simulink model "f_cd_reorder"  (R2018a)
settings: Solver=VariableStepAuto  StartTime=0.0  StopTime=200000  RelTol=1e-3
libraries: xbsIndex_r4 x1711, casper_library_misc x12, xps_library x2, simulink x1
(part 1 of 9)
settings Model: Creator=andrew  LastModifiedBy=andrew

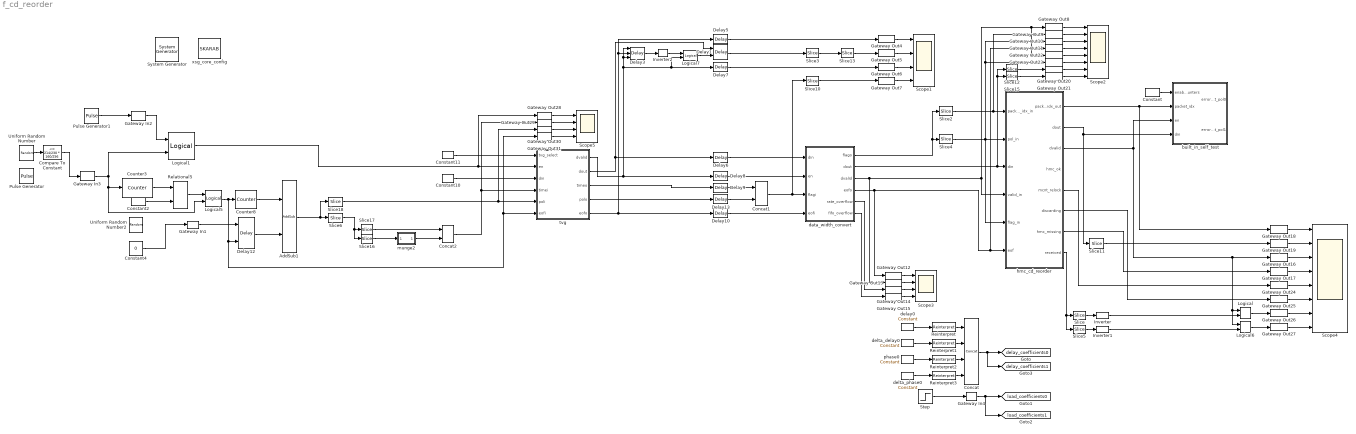
== system f_cd_reorder ==
  " System Generator" : xbsIndex_r4/ System Generator  Tag=genX  xilinxfamily=virtex7  part=xc7vx690t  speed=-2  package=ffg1927  synthesis_tool=XST  clock_wrapper=Clock Enables  directory=/home/skarab_fpga/source/feng_wide/s_c856m1k/sysgen  proj_type=Vivado  Synth_file=Vivado Synthesis Defaults  Impl_file=Vivado Implementation Defaults  testbench=off  simulink_period=1  sysclk_period=4.2017  dcm_input_clock_period=10  incr_netlist=off  trim_vbits=Everywhere in SubSystem  dbl_ovrd=According to Block Masks  core_generation=According to Block Masks  run_coregen=off  deprecated_control=off  eval_field=0  block_type=sysgen
  AddSub1 : xbsIndex_r4/AddSub  mode=Addition  use_carryin=off  use_carryout=off  en=off  latency=0  precision=User Defined  arith_type=Unsigned  n_bits=36+1  bin_pt=0  quantization=Truncate  overflow=Wrap  use_behavioral_HDL=off  hw_selection=Fabric  pipelined=off  dbl_ovrd=off  block_type=addsub
  Compare To Constant : simulink/Logic and Bit Operations/Compare To Constant  relop=<=  const=214/230 * 160/256  OutDataTypeStr=boolean
  Concat : xbsIndex_r4/Concat  num_inputs=4  dbl_ovrd=off  block_type=concat
  Concat1 : xbsIndex_r4/Concat  num_inputs=2  dbl_ovrd=off  block_type=concat
  Concat2 : xbsIndex_r4/Concat  num_inputs=2  dbl_ovrd=off  block_type=concat
  Constant : xbsIndex_r4/Constant  const=1  gui_display_data_type=Boolean  arith_type=Boolean  n_bits=1  bin_pt=0  preci_type=Single  exp_width=8  frac_width=24  explicit_period=on  period=1  equ=P=C  opselect=C  inp2=PCIN>>17  opr=+  inp1=P  carry=CIN  dbl_ovrd=off  block_type=constant
  Constant10 : xbsIndex_r4/Constant  const=0  gui_display_data_type=Fixed-point  arith_type=Unsigned  n_bits=256  bin_pt=0  preci_type=Single  exp_width=8  frac_width=24  explicit_period=on  period=1  equ=P=C  opselect=C  inp2=PCIN>>17  opr=+  inp1=P  carry=CIN  dbl_ovrd=off  block_type=constant
  Constant11 : xbsIndex_r4/Constant  const=1  gui_display_data_type=Fixed-point  arith_type=Unsigned  n_bits=1  bin_pt=0  preci_type=Single  exp_width=8  frac_width=24  explicit_period=on  period=1  equ=P=C  opselect=C  inp2=PCIN>>17  opr=+  inp1=P  carry=CIN  dbl_ovrd=off  block_type=constant
  Constant2 : xbsIndex_r4/Constant  const=(4096*10)/256-1  gui_display_data_type=Fixed-point  arith_type=Unsigned  n_bits=ceil(log2((4096*10)/256))  bin_pt=0  preci_type=Single  exp_width=8  frac_width=24  explicit_period=on  period=1  equ=P=C  opselect=C  inp2=PCIN>>17  opr=+  inp1=P  carry=CIN  dbl_ovrd=off  block_type=constant
  Constant4 : Constant  Value=0
  Counter3 : xbsIndex_r4/Counter  cnt_type=Count Limited  cnt_to=((4096*10)/256)-1  operation=Up  start_count=0  cnt_by_val=1  arith_type=Unsigned  n_bits=ceil(log2((4096*10)/256))  bin_pt=0  load_pin=off  rst=off  en=on  explicit_period=on  period=1  use_behavioral_HDL=off  implementation=Fabric  dbl_ovrd=off  block_type=counter
  Counter8 : xbsIndex_r4/Counter  cnt_type=Free Running  cnt_to=48  operation=Up  start_count=0*167  cnt_by_val=1  arith_type=Unsigned  n_bits=36+1  bin_pt=0  load_pin=off  rst=off  en=on  explicit_period=on  period=1  use_behavioral_HDL=off  implementation=Fabric  dbl_ovrd=off  block_type=counter
  Delay1 : xbsIndex_r4/Delay  rst=off  infoeditControl=Selection of Reset will increase slice count due to use of real FFs and instead of SRLs  en=on  latency=1  reg_retiming=on  dbl_ovrd=off  block_type=delay
  Delay{5..10,13} (7 alike) : xbsIndex_r4/Delay  rst=off  infoeditControl=Selection of Reset will increase slice count due to use of real FFs and instead of SRLs  en=off  latency=1  reg_retiming=on  dbl_ovrd=off  block_type=delay
  Delay12 : xbsIndex_r4/Delay  rst=off  infoeditControl=Selection of Reset will increase slice count due to use of real FFs and instead of SRLs  en=on  latency=1  reg_retiming=off  dbl_ovrd=off  block_type=delay
  Delay3 : xbsIndex_r4/Delay  rst=on  infoeditControl=Selection of Reset will increase slice count due to use of real FFs and instead of SRLs  en=on  latency=1  reg_retiming=on  dbl_ovrd=off  block_type=delay
  Gateway In1 : xbsIndex_r4/Gateway In  gui_display_data_type=Fixed-point  arith_type="Signed  (2's comp)"  n_bits=9  bin_pt=0  preci_type=Single  exp_width=8  frac_width=24  rows=1  columns=1  quantization="Round  (unbiased: +/- Inf)"  overflow=Saturate  period=1  UseAsADC=off  ADCChannel='1'  interface=None  automatic_assignment=on  address_offset=hex2dec('00')  intf_name=''  intf_description=''  default_value=0  timing_constraint=None  locs_specified=off  LOCs={}  io_standard={}  inherit_from_input=off  hdl_port=on  dbl_ovrd=off  block_type=gatewayin
  Gateway In2 : xbsIndex_r4/Gateway In  gui_display_data_type=Boolean  arith_type=Boolean  n_bits=16  bin_pt=14  preci_type=Single  exp_width=8  frac_width=24  rows=1  columns=1  quantization="Round  (unbiased: +/- Inf)"  overflow=Saturate  period=1  UseAsADC=off  ADCChannel='1'  interface=None  automatic_assignment=on  address_offset=hex2dec('00')  intf_name=''  intf_description=''  default_value=0  timing_constraint=None  locs_specified=off  LOCs={}  io_standard={}  inherit_from_input=off  hdl_port=on  dbl_ovrd=off  block_type=gatewayin
  Gateway In3 : xbsIndex_r4/Gateway In  gui_display_data_type=Boolean  arith_type=Boolean  n_bits=16  bin_pt=14  preci_type=Single  exp_width=8  frac_width=24  rows=1  columns=1  quantization="Round  (unbiased: +/- Inf)"  overflow=Saturate  period=1  UseAsADC=off  ADCChannel='1'  interface=None  automatic_assignment=on  address_offset=hex2dec('00')  intf_name=''  intf_description=''  default_value=0  timing_constraint=None  locs_specified=off  LOCs={}  io_standard={}  inherit_from_input=off  hdl_port=on  dbl_ovrd=off  block_type=gatewayin
  Gateway In4 : xbsIndex_r4/Gateway In  gui_display_data_type=Boolean  arith_type=Boolean  n_bits=16  bin_pt=14  preci_type=Single  exp_width=8  frac_width=24  rows=1  columns=1  quantization="Round  (unbiased: +/- Inf)"  overflow=Saturate  period=1  UseAsADC=off  ADCChannel='1'  interface=None  automatic_assignment=on  address_offset=hex2dec('00')  intf_name=''  intf_description=''  default_value=0  timing_constraint=None  locs_specified=off  LOCs={}  io_standard={}  inherit_from_input=off  hdl_port=on  dbl_ovrd=off  block_type=gatewayin
  Gateway Out{4..31} (28 alike) : xbsIndex_r4/Gateway Out  inherit_from_input=off  hdl_port=off  rows=1  columns=1  UseAsDAC=off  DACChannel='1'  interface=None  automatic_assignment=on  address_offset=hex2dec('00')  intf_name=''  intf_description=''  timing_constraint=None  locs_specified=off  LOCs={}  io_standard={}  block_type=gatewayout
  Inverter : xbsIndex_r4/Inverter  en=off  latency=0  dbl_ovrd=off  block_type=inv
  Inverter1 : xbsIndex_r4/Inverter  en=off  latency=0  dbl_ovrd=off  block_type=inv
  Inverter2 : xbsIndex_r4/Inverter  en=off  latency=0  dbl_ovrd=off  block_type=inv
  Logical{,1,5..7} (5 alike) : xbsIndex_r4/Logical  logical_function=AND  inputs=2  en=off  latency=0  precision=Full  arith_type=Unsigned  n_bits=16  bin_pt=0  align_bp=on  dbl_ovrd=off  block_type=logical
  Pulse Generator : DiscretePulseGenerator  Period=floor(256*(240/214))  PulseWidth=160  PhaseDelay=10
  Pulse Generator1 : DiscretePulseGenerator  Period=50000  PulseWidth=45000
  Reinterpret{,1..3} (4 alike) : xbsIndex_r4/Reinterpret  force_arith_type=on  arith_type=Unsigned  force_bin_pt=on  bin_pt=0  block_type=reinterpret
  Relational5 : xbsIndex_r4/Relational  mode=a=b  op_type=Bool  en=off  latency=0  dbl_ovrd=off  block_type=relational
  Scope1 : Scope  NumInputPorts=4
  Scope2 : Scope  NumInputPorts=8
  Scope3 : Scope  NumInputPorts=4
  Scope4 : Scope  NumInputPorts=8
  Scope5 : Scope  NumInputPorts=4
  Slice : xbsIndex_r4/Slice  nbits=1  boolean_output=on  mode=Upper Bit Location + Width  bit1=0  base1=MSB of Input  bit0=0  base0=LSB of Input  dbl_ovrd=off  block_type=slice
  Slice10 : xbsIndex_r4/Slice  nbits=49-12-1  boolean_output=off  mode=Upper Bit Location + Width  bit1=0  base1=MSB of Input  bit0=0  base0=LSB of Input  dbl_ovrd=off  block_type=slice
  Slice11 : xbsIndex_r4/Slice  nbits=80  boolean_output=off  mode=Upper Bit Location + Width  bit1=0  base1=MSB of Input  bit0=0  base0=LSB of Input  dbl_ovrd=off  block_type=slice
  Slice12 : xbsIndex_r4/Slice  nbits=80  boolean_output=off  mode=Upper Bit Location + Width  bit1=0  base1=MSB of Input  bit0=0  base0=LSB of Input  dbl_ovrd=off  block_type=slice
  Slice13 : xbsIndex_r4/Slice  nbits=36  boolean_output=off  mode=Lower Bit Location + Width  bit1=0  base1=MSB of Input  bit0=5+4+1  base0=LSB of Input  dbl_ovrd=off  block_type=slice
  Slice15 : xbsIndex_r4/Slice  nbits=80  boolean_output=off  mode=Lower Bit Location + Width  bit1=0  base1=MSB of Input  bit0=0  base0=LSB of Input  dbl_ovrd=off  block_type=slice
  Slice16 : xbsIndex_r4/Slice  nbits=10  boolean_output=off  mode=Lower Bit Location + Width  bit1=0  base1=MSB of Input  bit0=0  base0=LSB of Input  dbl_ovrd=off  block_type=slice
  Slice17 : xbsIndex_r4/Slice  nbits=8  boolean_output=off  mode=Two Bit Locations  bit1=0  base1=MSB of Input  bit0=10  base0=LSB of Input  dbl_ovrd=off  block_type=slice
  Slice18 : xbsIndex_r4/Slice  nbits=1  boolean_output=off  mode=Lower Bit Location + Width  bit1=0  base1=MSB of Input  bit0=0  base0=LSB of Input  dbl_ovrd=off  block_type=slice
  Slice2 : xbsIndex_r4/Slice  nbits=48-12  boolean_output=off  mode=Upper Bit Location + Width  bit1=0  base1=MSB of Input  bit0=0  base0=LSB of Input  dbl_ovrd=off  block_type=slice
  Slice3 : xbsIndex_r4/Slice  nbits=80  boolean_output=off  mode=Upper Bit Location + Width  bit1=0  base1=MSB of Input  bit0=0  base0=LSB of Input  dbl_ovrd=off  block_type=slice
  Slice4 : xbsIndex_r4/Slice  nbits=1  boolean_output=off  mode=Lower Bit Location + Width  bit1=0  base1=MSB of Input  bit0=0  base0=LSB of Input  dbl_ovrd=off  block_type=slice
  Slice5 : xbsIndex_r4/Slice  nbits=1  boolean_output=on  mode=Lower Bit Location + Width  bit1=0  base1=MSB of Input  bit0=0  base0=LSB of Input  dbl_ovrd=off  block_type=slice
  Slice6 : xbsIndex_r4/Slice  nbits=36  boolean_output=off  mode=Upper Bit Location + Width  bit1=0  base1=MSB of Input  bit0=0  base0=LSB of Input  dbl_ovrd=off  block_type=slice
  Step : Step  SampleTime=300
  Uniform Random Number : UniformRandomNumber  Minimum=0  SampleTime=1
  Uniform Random Number2 : UniformRandomNumber  Minimum=0  SampleTime=1
  built_in_self_test : Subsystem
  data_width_convert : Subsystem  mask{mux_latency=3, n_bits_din=256, n_bits_dout=160, max_burst_len=160*2}
      mask prompts: mux_latency "mux latency"; n_bits_din "data with in"; n_bits_dout "data width out"; max_burst_len "expected max input burst length"
      mask init:
      | %annotation = sprintf('latency=%i', mux_latency);
      | %set_param(gcb, 'AttributesFormatString', annotation);
      | annotation = sprintf('');
      | set_param(gcb, 'AttributesFormatString', annotation);
  delay0 : xbsIndex_r4/Constant  const=0  gui_display_data_type=Fixed-point  arith_type=Unsigned  n_bits=32  bin_pt=15  preci_type=Single  exp_width=8  frac_width=24  explicit_period=on  period=1  equ=P=C  opselect=C  inp2=PCIN>>17  opr=+  inp1=P  carry=CIN  dbl_ovrd=off  block_type=constant
  delta_delay0 : xbsIndex_r4/Constant  const=0  gui_display_data_type=Fixed-point  arith_type=Signed (2's comp)  n_bits=16  bin_pt=15  preci_type=Single  exp_width=8  frac_width=24  explicit_period=on  period=1  equ=P=C  opselect=C  inp2=PCIN>>17  opr=+  inp1=P  carry=CIN  dbl_ovrd=off  block_type=constant
  delta_phase0 : xbsIndex_r4/Constant  const=0  gui_display_data_type=Fixed-point  arith_type=Signed (2's comp)  n_bits=16  bin_pt=15  preci_type=Single  exp_width=8  frac_width=24  explicit_period=on  period=1  equ=P=C  opselect=C  inp2=PCIN>>17  opr=+  inp1=P  carry=CIN  dbl_ovrd=off  block_type=constant
  hmc_cd_reorder : Subsystem  mask{n_bits_max_delay=15, packet_size=256, n_bits_din=160, n_bits_sample=10, n_bits_flag=1, n_bits_timestamp=48 - 12, n_bits_fft=11}
      mask prompts: n_bits_max_delay "max sample delay required per pol (2^?)"; packet_size "words per packet"; n_bits_din "word bit width in"; n_bits_sample "sample bit width"; n_bits_flag "flag bit width in"; n_bits_timestamp "timestamp bit width"; n_bits_fft "fft size (2^?)"
      mask init:
      | n_bits_polarisations = 1;
      | double_buffer = 1; %we start reading once buffer half full so need to double buffer
      | n_bits_buffer_size = n_bits_max_delay+n_bits_polarisations+double_buffer;
      | packets = ((2^n_bits_buffer_size)*n_bits_sample)/(packet_size*n_bits_din);
      | n_bits_packets = ceil(log2(packets));
      | samples_per_word = n_bits_din/n_bits_sample;
      | samples_per_packet = (packet_size*n_bits_din)/n_bits_sample;
      | fmtstr = sprintf('Buffer space: \n%d packets per polarisation', floor(packets));
      | set_param(gcb, 'AttributesFormatString', fmtstr);
      settings: AttributesFormatString=|
      | Buffer space:
      | 32 packets per polarisation
  munge2 : Subsystem  AncestorBlock=casper_library_flow_control/munge  mask(munge){divisions=10, div_size=[1 1 1 1 1 1 1 1 1 1], order=[0 1 2 3 4 5 7 6 8 9], arith_type_out=Unsigned, bin_pt_out=0}
      mask prompts: divisions "Number of divisions"; div_size "Division size (bits)"; order "Division packing order"; arith_type_out "Output arithmetic type"; bin_pt_out "Output binary point"
      mask help: Splits an input bus into the specified number of divisions and then recombines them in the order specified (most significant division = 0,least = number divisions-1)
      mask init:
      | munge_init(gcb, ...
      |     'divisions', divisions, ...
      |     'div_size', div_size, ...
      |     'order', order, ...
      |     'arith_type_out', arith_type_out, ...
      |     'bin_pt_out', bin_pt_out);
      settings: AttributesFormatString=|
      | split:[1 1 1 1 1 1 1 1 1 1]
      | join:[0 1 2 3 4 5 7 6 8 9]
      | Unsigned [10,0]
      mask TypeOptions arith_type_out: Unsigned | Signed  (2's comp) | Floating-point
  phase0 : xbsIndex_r4/Constant  const=0  gui_display_data_type=Fixed-point  arith_type=Signed (2's comp)  n_bits=16  bin_pt=15  preci_type=Single  exp_width=8  frac_width=24  explicit_period=on  period=1  equ=P=C  opselect=C  inp2=PCIN>>17  opr=+  inp1=P  carry=CIN  dbl_ovrd=off  block_type=constant
  tvg : Subsystem
  xsg_core_config : xps_library/Platforms/SKARAB  Tag=xps:xsg  hw_sys=SKARAB:xc7vx690t  clk_src=sys_clk  clk_rate=238  sample_period=1  synthesis_tool=XST
      settings: SourceProductName=CASPER XPS Blockset
  tag scope: delay_coefficients0=global, delay_coefficients1=global, load_coefficients0=global, load_coefficients1=global
  wires:
  Gateway Out6/1 -> Scope1/3
  Gateway Out4/1 -> Scope1/1
  Gateway Out5/1 -> Scope1/2
  Slice3/1 -> Slice13/1
  Gateway Out7/1 -> Scope1/4
  Uniform Random Number/1 -> Compare To Constant/1
  data_width_convert/3(dvalid) -> Gateway Out22/1, Gateway Out8/1, hmc_cd_reorder/4(valid_in), Gateway Out13/1
  data_width_convert/4(eofo) -> Gateway Out11/1, hmc_cd_reorder/6(eof), Gateway Out12/1
  data_width_convert/1(flago) -> Slice2/1, Slice4/1
  Slice4/1 -> hmc_cd_reorder/5(flag_in), hmc_cd_reorder/2(pol_in), Gateway Out10/1, Gateway Out23/1
  Slice2/1 -> Gateway Out9/1, hmc_cd_reorder/1(packet_idx_in)
  Gateway Out11/1 -> Scope2/4
  Gateway Out9/1 -> Scope2/2
  Gateway Out8/1 -> Scope2/1
  Gateway Out10/1 -> Scope2/3
  data_width_convert/2(dout) -> Slice15/1, Slice12/1, hmc_cd_reorder/3(din)
  Delay5/1 -> Gateway Out4/1
  Concat1/1 -> data_width_convert/3(flagi), Slice10/1
  Delay7/1 -> Gateway Out6/1
  Slice10/1 -> Gateway Out7/1
  Delay6/1 -> data_width_convert/1(din)
  Delay8/1 -> data_width_convert/2(en)
  Delay10/1 -> data_width_convert/4(eofi)
  Gateway Out16/1 -> Scope4/3
  Gateway Out18/1 -> Scope4/1
  Gateway Out19/1 -> Scope4/2
  Gateway Out17/1 -> Scope4/4
  hmc_cd_reorder/1(packet_idx_out) -> built_in_self_test/2(packet_idx), Gateway Out18/1
  hmc_cd_reorder/3(dvalid) -> built_in_self_test/3(en), Logical/1, Logical6/1, Gateway Out16/1
  Slice11/1 -> Gateway Out19/1
  Gateway Out22/1 -> Scope2/5
  Gateway Out23/1 -> Scope2/6
  Gateway Out20/1 -> Scope2/7
  Gateway Out21/1 -> Scope2/8
  Slice12/1 -> Gateway Out20/1
  Slice15/1 -> Gateway Out21/1
  Gateway Out24/1 -> Scope4/5
  Gateway Out25/1 -> Scope4/6
  hmc_cd_reorder/7(hmc_missing) -> Gateway Out17/1
  hmc_cd_reorder/5(mcnt_relock) -> Gateway Out24/1
  hmc_cd_reorder/6(discarding) -> Gateway Out25/1
  hmc_cd_reorder/8(received) -> Slice5/1, Slice/1
  Gateway Out26/1 -> Scope4/7
  Gateway Out27/1 -> Scope4/8
  Delay12/1 -> AddSub1/2
  Gateway In1/1 -> Delay12/1
  AddSub1/1 -> Slice18/1, Slice6/1
  Counter8/1 -> AddSub1/1
  Slice6/1 -> Slice16/1, Slice17/1
  Slice17/1 -> Concat2/1
  Constant2/1 -> Relational5/2
  Counter3/1 -> Relational5/1
  Relational5/1 -> Logical5/1
  Logical5/1 -> Counter8/1, Gateway Out31/1, tvg/6(eofi), Delay12/2
  Gateway In3/1 -> Logical5/2, Counter3/1, Logical1/2
  Constant10/1 -> tvg/3(din)
  Slice18/1 -> Gateway Out30/1, tvg/5(poli)
  Constant11/1 -> tvg/1(tvg_select)
  tvg/2(dout) -> Delay1/1, Delay6/1
  tvg/1(dvalid) -> Delay8/1, Delay7/1, Logical7/2, Delay3/3, Delay3/1
  tvg/5(eofo) -> Delay10/1, Delay5/1, Delay3/2
  tvg/3(timeo) -> Delay9/1
  tvg/4(polo) -> Delay13/1
  Gateway Out31/1 -> Scope5/4
  Gateway Out30/1 -> Scope5/3
  Gateway Out29/1 -> Scope5/2
  Gateway Out28/1 -> Scope5/1
  Constant/1 -> built_in_self_test/1(enable_counters)
  hmc_cd_reorder/2(dout) -> Slice11/1, built_in_self_test/4(din)
  Delay13/1 -> Concat1/2
  Delay9/1 -> Concat1/1
  Gateway Out15/1 -> Scope3/4
  Gateway Out13/1 -> Scope3/2
  Gateway Out12/1 -> Scope3/1
  Gateway Out14/1 -> Scope3/3
  data_width_convert/5(rate_overflow) -> Gateway Out14/1
  data_width_convert/6(fifo_overflow) -> Gateway Out15/1
  Slice5/1 -> Inverter1/1
  Slice/1 -> Inverter/1
  Inverter/1 -> Logical/2
  Inverter1/1 -> Logical6/2
  Logical/1 -> Gateway Out26/1
  Logical6/1 -> Gateway Out27/1
  Concat2/1 -> Gateway Out29/1, tvg/4(timei)
  Compare To Constant/1 -> Gateway In3/1
  Reinterpret/1 -> Concat/1
  Reinterpret1/1 -> Concat/2
  Reinterpret2/1 -> Concat/3
  Reinterpret3/1 -> Concat/4
  delta_phase0/1 -> Reinterpret3/1
  phase0/1 -> Reinterpret2/1
  delta_delay0/1 -> Reinterpret1/1
  delay0/1 -> Reinterpret/1
  Concat/1 -> [delay_coefficients1], [delay_coefficients0]
  Step/1 -> Gateway In4/1
  Gateway In4/1 -> [load_coefficients1], [load_coefficients0]
  Slice16/1 -> munge2/1(din)
  Slice13/1 -> Gateway Out5/1
  Delay3/1 -> Inverter2/1
  Inverter2/1 -> Logical7/1
  Logical7/1 -> Delay1/2
  Delay1/1 -> Slice3/1
  Pulse Generator1/1 -> Gateway In2/1
  Gateway In2/1 -> Logical1/1
  Logical1/1 -> tvg/2(en), Gateway Out28/1
  Constant4/1 -> Gateway In1/1
  munge2/1(dout) -> Concat2/2

== system f_cd_reorder/built_in_self_test ==
  enable_counters : Inport
  packet_idx : Inport  Port=2
  en : Inport  Port=3
  din : Inport  Port=4
  Concat : xbsIndex_r4/Concat  num_inputs=3  dbl_ovrd=off  block_type=concat
  Concat1 : xbsIndex_r4/Concat  num_inputs=2  dbl_ovrd=off  block_type=concat
  Concat2 : xbsIndex_r4/Concat  num_inputs=2  dbl_ovrd=off  block_type=concat
  Constant : xbsIndex_r4/Constant  const=0  gui_display_data_type=Fixed-point  arith_type=Unsigned  n_bits=1  bin_pt=0  preci_type=Single  exp_width=8  frac_width=24  explicit_period=on  period=1  equ=P=C  opselect=C  inp2=PCIN>>17  opr=+  inp1=P  carry=CIN  dbl_ovrd=off  block_type=constant
  Constant1 : xbsIndex_r4/Constant  const=1  gui_display_data_type=Fixed-point  arith_type=Unsigned  n_bits=1  bin_pt=0  preci_type=Single  exp_width=8  frac_width=24  explicit_period=on  period=1  equ=P=C  opselect=C  inp2=PCIN>>17  opr=+  inp1=P  carry=CIN  dbl_ovrd=off  block_type=constant
  Constant2 : xbsIndex_r4/Constant  const=0  gui_display_data_type=Fixed-point  arith_type=Unsigned  n_bits=2  bin_pt=0  preci_type=Single  exp_width=8  frac_width=24  explicit_period=on  period=1  equ=P=C  opselect=C  inp2=PCIN>>17  opr=+  inp1=P  carry=CIN  dbl_ovrd=off  block_type=constant
  Counter : xbsIndex_r4/Counter  cnt_type=Free Running  cnt_to=Inf  operation=Up  start_count=0  cnt_by_val=1  arith_type=Unsigned  n_bits=12-3  bin_pt=0  load_pin=off  rst=on  en=on  explicit_period=on  period=1  use_behavioral_HDL=off  implementation=Fabric  dbl_ovrd=off  block_type=counter
  Delay{,1..4} (5 alike) : xbsIndex_r4/Delay  rst=off  infoeditControl=Selection of Reset will increase slice count due to use of real FFs and instead of SRLs  en=off  latency=1  reg_retiming=on  dbl_ovrd=off  block_type=delay
  Delay{5..8} (4 alike) : xbsIndex_r4/Delay  rst=off  infoeditControl=Selection of Reset will increase slice count due to use of real FFs and instead of SRLs  en=off  latency=1  reg_retiming=off  dbl_ovrd=off  block_type=delay
  Gateway Out{,1..7} (8 alike) : xbsIndex_r4/Gateway Out  inherit_from_input=off  hdl_port=off  rows=1  columns=1  UseAsDAC=off  DACChannel='1'  interface=None  automatic_assignment=on  address_offset=hex2dec('00')  intf_name=''  intf_description=''  timing_constraint=None  locs_specified=off  LOCs={}  io_standard={}  block_type=gatewayout
  Inverter : xbsIndex_r4/Inverter  en=off  latency=0  dbl_ovrd=off  block_type=inv
  Logical : xbsIndex_r4/Logical  logical_function=AND  inputs=2  en=off  latency=1  precision=Full  arith_type=Unsigned  n_bits=16  bin_pt=0  align_bp=on  dbl_ovrd=off  block_type=logical
  Logical1 : xbsIndex_r4/Logical  logical_function=AND  inputs=2  en=off  latency=1  precision=Full  arith_type=Unsigned  n_bits=16  bin_pt=0  align_bp=on  dbl_ovrd=off  block_type=logical
  Relational : xbsIndex_r4/Relational  mode=a!=b  op_type=Bool  en=off  latency=0  dbl_ovrd=off  block_type=relational
  Relational1 : xbsIndex_r4/Relational  mode=a!=b  op_type=Bool  en=off  latency=0  dbl_ovrd=off  block_type=relational
  Relational2 : xbsIndex_r4/Relational  mode=a!=b  op_type=Bool  en=off  latency=0  dbl_ovrd=off  block_type=relational
  Scope : Scope  NumInputPorts=8
  Slice : xbsIndex_r4/Slice  nbits=80  boolean_output=off  mode=Upper Bit Location + Width  bit1=0  base1=MSB of Input  bit0=0  base0=LSB of Input  dbl_ovrd=off  block_type=slice
  Slice1 : xbsIndex_r4/Slice  nbits=80  boolean_output=off  mode=Lower Bit Location + Width  bit1=0  base1=MSB of Input  bit0=0  base0=LSB of Input  dbl_ovrd=off  block_type=slice
  Slice2 : xbsIndex_r4/Slice  nbits=48  boolean_output=off  mode=Lower Bit Location + Width  bit1=0  base1=MSB of Input  bit0=0  base0=LSB of Input  dbl_ovrd=off  block_type=slice
  Slice3 : xbsIndex_r4/Slice  nbits=48  boolean_output=off  mode=Lower Bit Location + Width  bit1=0  base1=MSB of Input  bit0=0  base0=LSB of Input  dbl_ovrd=off  block_type=slice
  error_counter0 : xbsIndex_r4/Counter  cnt_type=Free Running  cnt_to=Inf  operation=Up  start_count=0  cnt_by_val=1  arith_type=Unsigned  n_bits=8  bin_pt=0  load_pin=off  rst=on  en=on  explicit_period=on  period=1  use_behavioral_HDL=off  implementation=Fabric  dbl_ovrd=off  block_type=counter
  error_counter1 : xbsIndex_r4/Counter  cnt_type=Free Running  cnt_to=Inf  operation=Up  start_count=0  cnt_by_val=1  arith_type=Unsigned  n_bits=8  bin_pt=0  load_pin=off  rst=on  en=on  explicit_period=on  period=1  use_behavioral_HDL=off  implementation=Fabric  dbl_ovrd=off  block_type=counter
  error_cnt_pol0 : Outport
  error_cnt_pol1 : Outport  Port=2
  wires:
  enable_counters/1 -> Inverter/1
  Inverter/1 -> error_counter1/1, error_counter0/1
  error_counter0/1 -> Gateway Out6/1, error_cnt_pol0/1
  error_counter1/1 -> error_cnt_pol1/1, Gateway Out7/1
  en/1 -> Delay7/1
  packet_idx/1 -> Relational2/2, Delay5/1, Delay6/1
  Gateway Out/1 -> Scope/1
  din/1 -> Delay8/1
  Gateway Out1/1 -> Scope/2
  Slice/1 -> Slice3/1
  Concat/1 -> Concat2/1, Concat1/1
  Gateway Out2/1 -> Scope/3
  Gateway Out3/1 -> Scope/4
  Constant/1 -> Concat1/2
  Concat1/1 -> Relational/1, Delay3/1
  Constant1/1 -> Concat2/2
  Slice1/1 -> Slice2/1
  Concat2/1 -> Relational1/1
  Logical1/1 -> error_counter1/2
  Relational/1 -> Logical/2, Delay4/1
  Relational1/1 -> Logical1/2
  Gateway Out4/1 -> Scope/5
  Logical/1 -> Gateway Out5/1, error_counter0/2
  Gateway Out5/1 -> Scope/6
  Delay/1 -> Gateway Out/1
  Delay1/1 -> Gateway Out1/1
  Delay2/1 -> Gateway Out2/1
  Delay3/1 -> Gateway Out3/1
  Delay4/1 -> Gateway Out4/1
  Gateway Out6/1 -> Scope/7
  Delay5/1 -> Relational2/1
  Relational2/1 -> Delay1/1, Counter/1
  Delay7/1 -> Logical1/1, Logical/1, Delay/1, Counter/2
  Delay8/1 -> Slice1/1, Slice/1
  Counter/1 -> Concat/3
  Slice2/1 -> Relational1/2
  Slice3/1 -> Relational/2, Delay2/1
  Gateway Out7/1 -> Scope/8
  Delay6/1 -> Concat/2
  Constant2/1 -> Concat/1

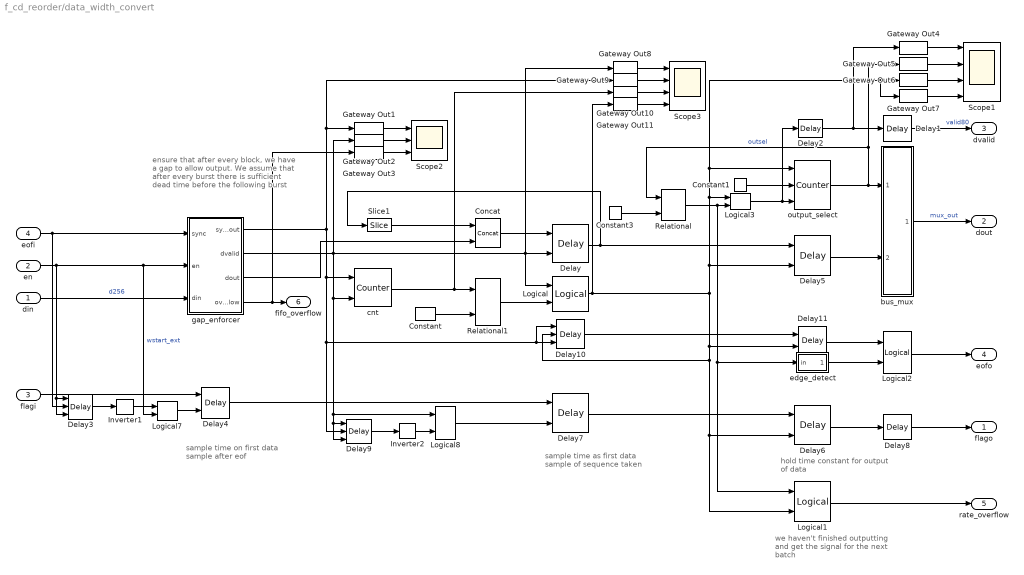
== system f_cd_reorder/data_width_convert ==
  note: ensure that after every
      | block, we have a gap to
      | allow output. We assume that
      | after every burst there is sufficient
      | dead time before the following burst
  note: we haven't finished
      | outputting and get
      | the signal for the next
      | batch
  note: sample time as
      | first data sample of
      | sequence taken
  note: hold time constant
      | for output of data
  note: sample time on
      | first data sample
      | after eof
  din : Inport
  en : Inport  Port=2
  flagi : Inport  Port=3
  eofi : Inport  Port=4
  Concat : xbsIndex_r4/Concat  num_inputs=2  dbl_ovrd=off  block_type=concat
  Constant : xbsIndex_r4/Constant  const=lcm(n_bits_din, n_bits_dout)/n_bits_din-1  gui_display_data_type=Fixed-point  arith_type=Unsigned  n_bits=ceil(log2(lcm(n_bits_din, n_bits_dout)/n_bits_din))  bin_pt=0  preci_type=Single  exp_width=8  frac_width=24  explicit_period=on  period=1  equ=P=C  opselect=C  inp2=PCIN>>17  opr=+  inp1=P  carry=CIN  dbl_ovrd=off  block_type=constant
  Constant1 : xbsIndex_r4/Constant  const=0  gui_display_data_type=Fixed-point  arith_type=Unsigned  n_bits=ceil(log2(lcm(n_bits_din, n_bits_dout)/n_bits_dout))  bin_pt=0  preci_type=Single  exp_width=8  frac_width=24  explicit_period=on  period=1  equ=P=C  opselect=C  inp2=PCIN>>17  opr=+  inp1=P  carry=CIN  dbl_ovrd=off  block_type=constant
  Constant3 : xbsIndex_r4/Constant  const=(lcm(n_bits_din, n_bits_dout)/n_bits_dout)-1  gui_display_data_type=Fixed-point  arith_type=Unsigned  n_bits=ceil(log2(lcm(n_bits_din, n_bits_dout)/n_bits_dout))  bin_pt=0  preci_type=Single  exp_width=8  frac_width=24  explicit_period=on  period=1  equ=P=C  opselect=C  inp2=PCIN>>17  opr=+  inp1=P  carry=CIN  dbl_ovrd=off  block_type=constant
  Delay{,4..7,11} (6 alike) : xbsIndex_r4/Delay  rst=off  infoeditControl=Selection of Reset will increase slice count due to use of real FFs and instead of SRLs  en=on  latency=1  reg_retiming=on  dbl_ovrd=off  block_type=delay
  Delay1 : xbsIndex_r4/Delay  rst=off  infoeditControl=Selection of Reset will increase slice count due to use of real FFs and instead of SRLs  en=off  latency=mux_latency  reg_retiming=on  dbl_ovrd=off  block_type=delay
  Delay10 : xbsIndex_r4/Delay  rst=on  infoeditControl=Selection of Reset will increase slice count due to use of real FFs and instead of SRLs  en=on  latency=1  reg_retiming=on  dbl_ovrd=off  block_type=delay
  Delay2 : xbsIndex_r4/Delay  rst=off  infoeditControl=Selection of Reset will increase slice count due to use of real FFs and instead of SRLs  en=off  latency=1  reg_retiming=on  dbl_ovrd=off  block_type=delay
  Delay3 : xbsIndex_r4/Delay  rst=on  infoeditControl=Selection of Reset will increase slice count due to use of real FFs and instead of SRLs  en=on  latency=1  reg_retiming=on  dbl_ovrd=off  block_type=delay
  Delay8 : xbsIndex_r4/Delay  rst=off  infoeditControl=Selection of Reset will increase slice count due to use of real FFs and instead of SRLs  en=off  latency=mux_latency  reg_retiming=on  dbl_ovrd=off  block_type=delay
  Delay9 : xbsIndex_r4/Delay  rst=on  infoeditControl=Selection of Reset will increase slice count due to use of real FFs and instead of SRLs  en=on  latency=1  reg_retiming=on  dbl_ovrd=off  block_type=delay
  Gateway Out{1..11} (11 alike) : xbsIndex_r4/Gateway Out  inherit_from_input=off  hdl_port=off  rows=1  columns=1  UseAsDAC=off  DACChannel='1'  interface=None  automatic_assignment=on  address_offset=hex2dec('00')  intf_name=''  intf_description=''  timing_constraint=None  locs_specified=off  LOCs={}  io_standard={}  block_type=gatewayout
  Inverter1 : xbsIndex_r4/Inverter  en=off  latency=0  dbl_ovrd=off  block_type=inv
  Inverter2 : xbsIndex_r4/Inverter  en=off  latency=0  dbl_ovrd=off  block_type=inv
  Logical : xbsIndex_r4/Logical  logical_function=AND  inputs=2  en=off  latency=1  precision=Full  arith_type=Unsigned  n_bits=16  bin_pt=0  align_bp=on  dbl_ovrd=off  block_type=logical
  Logical1 : xbsIndex_r4/Logical  logical_function=AND  inputs=2  en=off  latency=1  precision=Full  arith_type=Unsigned  n_bits=16  bin_pt=0  align_bp=on  dbl_ovrd=off  block_type=logical
  Logical2 : xbsIndex_r4/Logical  logical_function=AND  inputs=2  en=off  latency=3  precision=Full  arith_type=Unsigned  n_bits=16  bin_pt=0  align_bp=on  dbl_ovrd=off  block_type=logical
  Logical3 : xbsIndex_r4/Logical  logical_function=OR  inputs=2  en=off  latency=0  precision=Full  arith_type=Unsigned  n_bits=16  bin_pt=0  align_bp=on  dbl_ovrd=off  block_type=logical
  Logical7 : xbsIndex_r4/Logical  logical_function=AND  inputs=2  en=off  latency=0  precision=Full  arith_type=Unsigned  n_bits=16  bin_pt=0  align_bp=on  dbl_ovrd=off  block_type=logical
  Logical8 : xbsIndex_r4/Logical  logical_function=AND  inputs=2  en=off  latency=0  precision=Full  arith_type=Unsigned  n_bits=16  bin_pt=0  align_bp=on  dbl_ovrd=off  block_type=logical
  Relational : xbsIndex_r4/Relational  mode=a<b  op_type=Bool  en=off  latency=0  dbl_ovrd=off  block_type=relational
  Relational1 : xbsIndex_r4/Relational  mode=a=b  op_type=Bool  en=off  latency=0  dbl_ovrd=off  block_type=relational
  Scope1 : Scope  NumInputPorts=4
  Scope2 : Scope  NumInputPorts=3
  Scope3 : Scope  NumInputPorts=4
  Slice1 : xbsIndex_r4/Slice  nbits=lcm(n_bits_din, n_bits_dout)-n_bits_din  boolean_output=off  mode=Lower Bit Location + Width  bit1=0  base1=MSB of Input  bit0=0  base0=LSB of Input  dbl_ovrd=off  block_type=slice
  bus_mux : Subsystem  AncestorBlock=casper_library_bus/bus_mux  mask(bus_mux){n_inputs=1, n_bits=n_bits_dout * ones(1, lcm(n_bits_din, n_bits_dout)/n_bits_dout), cmplx=off, misc=off, mux_latency=mux_latency}
      mask prompts: n_inputs "number of inputs"; n_bits "input bit widths"; cmplx "complex data"; misc "misc support"; mux_latency "mux latency"
      mask help: Mux components of bus
      mask init:
      | bus_mux_init(gcb, ...
      |     'n_inputs', n_inputs, ...
      |     'n_bits', n_bits, ...
      |     'cmplx', cmplx, ...
      |     'misc', misc, ...
      |     'mux_latency', mux_latency);
  cnt : xbsIndex_r4/Counter  cnt_type=Count Limited  cnt_to=lcm(n_bits_din, n_bits_dout)/n_bits_din-1  operation=Up  start_count=0  cnt_by_val=1  arith_type=Unsigned  n_bits=ceil(log2(lcm(n_bits_din, n_bits_dout)/n_bits_din))  bin_pt=0  load_pin=off  rst=on  en=on  explicit_period=on  period=1  use_behavioral_HDL=on  implementation=Fabric  dbl_ovrd=off  block_type=counter
  edge_detect : Subsystem  AncestorBlock=casper_library_misc/edge_detect  mask(edge_detect){edge=Falling, polarity=Active High, x_in=[0 0.08 0.08 0.16 0.16 0.24 0.24 0.32 0.32 0.4], y_in=[-1 -1  1  1  1  1  1  1  1  1], x_out=[0.6 0.68 0.68 0.76 0.76 0.84 0.84 0.92 0.92 1], y_out=[-1 -1  1  1 -1 -1 -1 -1 -1 -1]}
      mask prompts: edge "Edge Type"; polarity "Output Polarity"; x_in "Input X Positions"; y_in "Input Y Positions"; x_out "Output X Positions"; y_out "Output Y Positions"
      mask help: Output is active for one-cycle after each edge of the specified type (i.e. rising, falling or both).
      mask init:
      | edge_detect_init(gcb,...
      |     'edge',edge,...
      |     'polarity',polarity,...
      |     'x_in',x_in,...
      |     'x_out',x_out,...
      |     'y_in',y_in,...
      |     'y_out',y_out);
      | 
      | x_in_num=str2num(getfield(getfield(get_param(gcb,'UserData'),'parameters'),'x_in'));
      | x_out_num=str2num(getfield(getfield(get_param(gcb,'UserData'),'parameters'),'x_out'));
      | y_in_num=str2num(getfield(getfield(get_param(gcb,'UserData'),'parameters'),'y_in'));
      | y_out_num=str2num(getfield(getfield(get_param(gcb,'UserData'),'parameters'),'y_out'));
      settings: AttributesFormatString=|
      | falling edges
      | active high
      mask Help: Output is active for one-cycle after each edge of the specified type (i.e. rising, falling, or both).  Latency is zero.
      mask TypeOptions edge: Rising | Falling | Both
      mask TypeOptions polarity: Active High | Active Low
      mask Display:
      | plot(x_in_num,0.5+y_in_num*0.2);
      | plot(x_out_num,0.5+y_out_num*0.2);
  gap_enforcer : Subsystem  mask{block_size=lcm(n_bits_din, n_bits_dout)/n_bits_din, gap_size=lcm(n_bits_din, n_bits_dout)/n_bits_dout - lcm(n_bits_din, n_bits_dout)/n_bits_din, max_burst_len=max_burst_len}
      mask prompts: block_size "data block size"; gap_size "gap size"; max_burst_len "max burst length"
      mask init:
      | set_param([gcb,'/fifo'], 'depth', num2str(2^(ceil(log2(max_burst_len)))));
  output_select : xbsIndex_r4/Counter  cnt_type=Free Running  cnt_to=Inf  operation=Up  start_count=(lcm(n_bits_din, n_bits_dout)/n_bits_dout)-1  cnt_by_val=1  arith_type=Unsigned  n_bits=ceil(log2(lcm(n_bits_din, n_bits_dout)/n_bits_dout))  bin_pt=0  load_pin=on  rst=off  en=on  explicit_period=on  period=1  use_behavioral_HDL=on  implementation=Fabric  dbl_ovrd=off  block_type=counter
  flago : Outport
  dout : Outport  Port=2
  dvalid : Outport  Port=3
  eofo : Outport  Port=4
  rate_overflow : Outport  Port=5
  fifo_overflow : Outport  Port=6
  wires:
  bus_mux/1(out) -> dout/1  "mux_out"
  output_select/1 -> Gateway Out5/1, Relational/1, bus_mux/1(sel)  "outsel"
  Delay1/1 -> dvalid/1  "valid80"
  en/1 -> Logical7/2, gap_enforcer/2(en), Delay3/3, Delay3/1  "wstart_ext"
  Delay8/1 -> flago/1
  Concat/1 -> Delay/1
  cnt/1 -> Gateway Out10/1, Relational1/1
  Constant/1 -> Relational1/2
  Relational1/1 -> Logical/2
  Logical/1 -> Gateway Out11/1, Delay6/2, Logical1/2, Delay10/2, Delay11/2, Logical3/1, output_select/1, Gateway Out7/1, Gateway Out6/1, Delay5/2
  Delay/1 -> Slice1/1, Delay5/1
  Logical8/1 -> Delay7/2
  flagi/1 -> Delay4/1
  Delay6/1 -> Delay8/1
  Delay7/1 -> Delay6/1
  Logical1/1 -> rate_overflow/1
  Constant1/1 -> output_select/2
  Constant3/1 -> Relational/2
  Logical3/1 -> Delay2/1, output_select/3
  Relational/1 -> edge_detect/1(in), Logical1/1, Logical3/2
  Delay2/1 -> Gateway Out4/1, Delay1/1
  Slice1/1 -> Concat/1
  Gateway Out4/1 -> Scope1/1
  Gateway Out5/1 -> Scope1/2
  Gateway Out6/1 -> Scope1/3
  Gateway Out7/1 -> Scope1/4
  din/1 -> gap_enforcer/3(din)  "d256"
  eofi/1 -> Delay3/2, gap_enforcer/1(sync)
  gap_enforcer/2(dvalid) -> Gateway Out2/1, Gateway Out8/1, Delay/2, Logical/1, Delay9/1, Delay9/3, Logical8/1, cnt/2
  Delay3/1 -> Inverter1/1
  Logical7/1 -> Delay4/2
  Delay4/1 -> Delay7/1
  Inverter1/1 -> Logical7/1
  Delay9/1 -> Inverter2/1
  Inverter2/1 -> Logical8/2
  Gateway Out2/1 -> Scope2/2
  Gateway Out1/1 -> Scope2/1
  gap_enforcer/3(dout) -> Concat/2
  gap_enforcer/1(sync_out) -> Delay9/2, Delay10/1, Delay10/3, cnt/1, Gateway Out9/1, Gateway Out1/1
  gap_enforcer/4(overflow) -> Gateway Out3/1, fifo_overflow/1
  Gateway Out3/1 -> Scope2/3
  Delay10/1 -> Delay11/1
  Logical2/1 -> eofo/1
  Delay11/1 -> Logical2/1
  edge_detect/1(out) -> Logical2/2
  Gateway Out10/1 -> Scope3/3
  Gateway Out8/1 -> Scope3/1
  Gateway Out9/1 -> Scope3/2
  Gateway Out11/1 -> Scope3/4
  Delay5/1 -> bus_mux/2(d0)
